simulink model "convertidor_pid_electrolizador"  (R2021a)
settings: Solver=VariableStepAuto  StartTime=0.0  StopTime=10  RelTol=1e-1
undefined symbols (not defined in the file): magnitude
libraries: spsSeriesRLCBranchLib x9, spsCurrentMeasurementLib x3, spsDiodeLib x3, simulink x3, spsGroundLib x2, spsMosfetLib x2, spsControlledVoltageSourceLib x1, pid_lib x1, spsDCVoltageSourceLib x1, spsVoltageMeasurementLib x1, spspowerguiLib x1
settings Model: Creator=Usuario  LastModifiedBy=Usuario

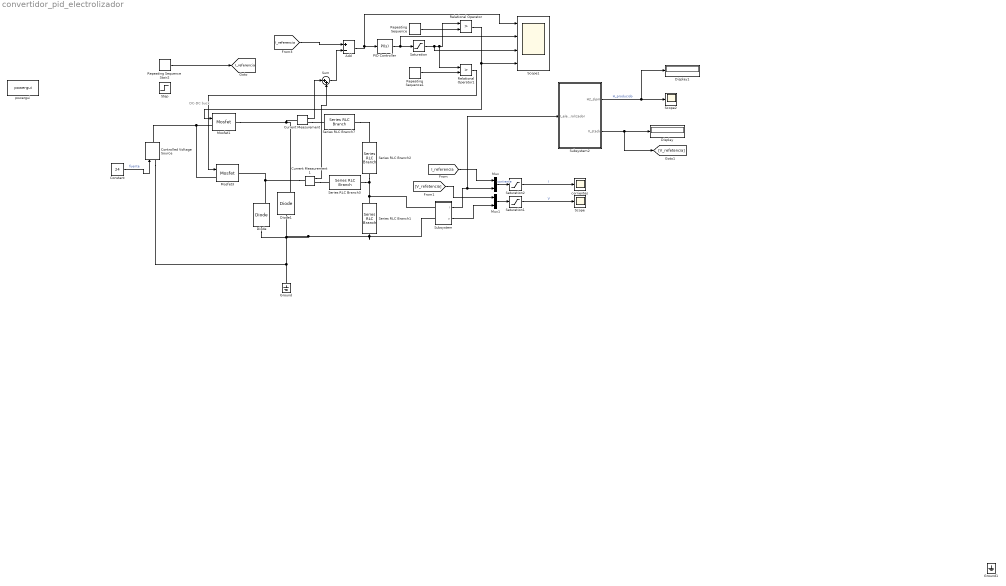
== system convertidor_pid_electrolizador ==
  note: DC-DC buck
  Add : Sum  Inputs=+-
  Constant : Constant  Value=24
  Controlled Voltage Source : spsControlledVoltageSourceLib/Controlled Voltage Source  Initialize=on  Source_Type=DC  Amplitude=10  Phase=0  Frequency=0  Measurements=None
  Current Measurement : spsCurrentMeasurementLib/Current Measurement  PhasorSimulation=off  OutputType=Complex  PSBequivalent=0
  Current Measurement1 : spsCurrentMeasurementLib/Current Measurement  PhasorSimulation=off  OutputType=Complex  PSBequivalent=0
  Diode : spsDiodeLib/Diode  Ron=0.001  Lon=0  Vf=0.8  IC=0  UseSnubber=0  Rs=500  Cs=250e-9  Measurements=on
  Diode1 : spsDiodeLib/Diode  Ron=0.001  Lon=0  Vf=0.8  IC=0  UseSnubber=0  Rs=500  Cs=250e-9  Measurements=on
  Display : Display
  Display1 : Display
  Ground : spsGroundLib/Ground  LConnTagsString=a
  Ground1 : spsGroundLib/Ground  LConnTagsString=a
  Mosfet1 : spsMosfetLib/Mosfet  Ron=0.001  Lon=0  Rd=0.01  Vfd=0  IC=0  Rs=1e5  Cs=inf  Measurements=off
  Mosfet3 : spsMosfetLib/Mosfet  Ron=0.001  Lon=0  Rd=0.01  Vfd=0  IC=0  Rs=1e5  Cs=inf  Measurements=off
  Mux : Mux  Inputs=2
  Mux1 : Mux  Inputs=2
  PID Controller : pid_lib/PID Controller  Controller=PI  Form=Parallel  TimeDomain=Continuous-time  UseExternalTs=off  SampleTime=-1  IntegratorMethod=Forward Euler  FilterMethod=Forward Euler  ControllerParametersSource=internal  P=7.85  I=261.799  D=1  UseFilter=on  N=1436119.989540  TunerSelectOption=Transfer Function Based (PID Tuner App)  InitialConditionSource=internal  InitialConditionForIntegrator=0  InitialConditionForFilter=0  DifferentiatorICPrevScaledInput=0  ExternalReset=none  TrackingMode=off  Kt=1  LimitOutput=off  SatLimitsSource=internal  UpperSaturationLimit=inf  LowerSaturationLimit=-inf  LinearizeAsGain=on  AntiWindupMode=none  Kb=1  POutMin=[]  POutMax=[]  IOutMin=[]  IOutMax=[]  DOutMin=[]  DOutMax=[]  NOutMin=[]  NOutMax=[]  SumOutMin=[]  SumOutMax=[]  SaturationOutMin=[]  SaturationOutMax=[]  PParamMin=[]  PParamMax=[]  IParamMin=[]  IParamMax=[]  DParamMin=[]  DParamMax=[]  NParamMin=[]  NParamMax=[]  KbParamMin=[]  KbParamMax=[]  KtParamMin=[]  KtParamMax=[]  KbOutMin=[]  KbOutMax=[]  KtOutMin=[]  KtOutMax=[]  IntegratorOutMin=[]  IntegratorOutMax=[]  FilterOutMin=[]  FilterOutMax=[]  SumI1OutMin=[]  SumI1OutMax=[]  SumI2OutMin=[]  SumI2OutMax=[]  SumI3OutMin=[]  SumI3OutMax=[]  SumI4OutMin=[]  SumI4OutMax=[]  SumDOutMin=[]  SumDOutMax=[]  DifferentiatorOutMin=[]  DifferentiatorOutMax=[]  FilterDiffOutCoefMin=[]  FilterDiffOutCoefMax=[]  ReciprocalOutMin=[]  ReciprocalOutMax=[]  SumDenOutMin=[]  SumDenOutMax=[]  SumNumOutMin=[]  SumNumOutMax=[]  DivideOutMin=[]  DivideOutMax=[]  UdiffTsProdOutMin=[]  UdiffTsProdOutMax=[]  NTsProdOutMin=[]  NTsProdOutMax=[]  UintegralTsProdOutMin=[]  UintegralTsProdOutMax=[]  UngainTsProdOutMin=[]  UngainTsProdOutMax=[]  IntegratorContinuousStateAttributes=''  IntegratorStateMustResolveToSignalObject=off  IntegratorRTWStateStorageClass=Auto  FilterContinuousStateAttributes=''  FilterStateMustResolveToSignalObject=off  FilterRTWStateStorageClass=Auto  ParallelPVariant=InternalParameters  IdealPVariant=Disabled  IVariant=InternalParameters  DVariant=Disabled  IntegratorVariant=Continuous  SatVariant=Disabled  AWVariant=Passthrough  PCopyVariant=Disabled  TRVariant=Disabled  FdbkBlocksVariant=Forward  IdealPFdbkVariant=Disabled  SatFdbkVariant=Disabled  DerivativeFilterVariant=Disabled  NVariant=Disabled  NCopyVariant=Disabled_SignalSpec  FilterICVariant=Disabled  IntegratorICVariant=InternalICs  ExternalResetVariant=Disabled  TRSumVariant=Passthrough  SumFdbkVariant=Disabled  SumVariant=Sum_PI  TsampFilterVariant=InternalTs  TsampNgainVariant=Passthrough  TsampIntegralVariant=Passthrough  ExternalSaturationOutDataTypeStr=Inherit: Same as second input
  Relational Operator : RelationalOperator  Operator=>  OutDataTypeStr=boolean  RndMeth=Simplest
  Relational Operator1 : RelationalOperator  Operator=>  OutDataTypeStr=boolean  RndMeth=Simplest
  Repeating Sequence : simulink/Sources/Repeating Sequence  rep_seq_t=[0 0.0001]  rep_seq_y=[0 1]
  Repeating Sequence Stair2 : simulink/Sources/Repeating Sequence Stair  OutValues=[0.1 10 40 19 20.8]  tsamp=2  OutMin=[]  OutMax=[]  OutDataTypeStr=double  OutputDataTypeScalingMode=double  OutDataType=fixdt(0,8)  ConRadixGroup=Best Precision: Vector-wise  OutScaling=2^-12
  Repeating Sequence1 : simulink/Sources/Repeating Sequence  rep_seq_t=[0 0.0001]  rep_seq_y=[1 0]
  Saturation : Saturate  UpperLimit=0.95  LowerLimit=0.01
  Saturation1 : Saturate  UpperLimit=19  LowerLimit=0
  Saturation2 : Saturate  UpperLimit=100  LowerLimit=0
  Scope : Scope
  Scope1 : Scope  NumInputPorts=4
  Scope2 : Scope
  Series RLC Branch1 : spsSeriesRLCBranchLib/Series RLC Branch  LConnTagsString=__new0  RConnTagsString=__new0  BranchType=C  Resistance=0.01  Inductance=1e-3  SetiL0=off  InitialCurrent=0  Capacitance=21.55e-6  Setx0=off  InitialVoltage=0  Measurements=None
  Series RLC Branch2 : spsSeriesRLCBranchLib/Series RLC Branch  LConnTagsString=__new0  RConnTagsString=__new0  BranchType=C  Resistance=0.01  Inductance=1e-3  SetiL0=off  InitialCurrent=0  Capacitance=21.55e-6  Setx0=off  InitialVoltage=0  Measurements=None
  Series RLC Branch3 : spsSeriesRLCBranchLib/Series RLC Branch  LConnTagsString=__new0  RConnTagsString=__new0  BranchType=L  Resistance=0.001  Inductance=299.6e-6  SetiL0=off  InitialCurrent=0  Capacitance=1e-6  Setx0=off  InitialVoltage=0  Measurements=None
  Series RLC Branch7 : spsSeriesRLCBranchLib/Series RLC Branch  LConnTagsString=__new0  RConnTagsString=__new0  BranchType=L  Resistance=0.001  Inductance=299.6e-6  SetiL0=off  InitialCurrent=0  Capacitance=1e-6  Setx0=off  InitialVoltage=0  Measurements=None
  Step : Step  Time=0.5  After=40  SampleTime=0
  Subsystem : Subsystem
  Subsystem2 : Subsystem
  Sum : Sum  Inputs=|++
  corrientes : Scope
  powergui : spspowerguiLib/powergui  Priority=1  SimulationMode=Discrete  SampleTime=1e-5  frequency=60  Iterations=50  frequencyindice=0  Pbase=100e6  ErrMax=1e-4  UnitsV=kV  UnitsW=MW  buscounter=0  FunctionMessages=off  echomessages=off  EnableUseOfTLC=off  CurrentSourceSwitches=off  DisableSnubberDevices=off  DisableRonSwitches=off  DisableVfSwitches=off  DisplayEquations=off  AutomaticDiscreteSolvers=off  SolverType=Tustin/Backward Euler (TBE)  Interpol=off  ExternalGateDelay=off  methode=off  Ts=100  x0status=blocks  SPID=on  SwTol=0  HookPort=off  NonlinearTolerance=1e-4  nMaxIteration=100  ContinueOnMaxIteration=off  RestoreLinks=warning  ResistiveCurrentMeasurement=off  Frange=[0:2:500]  Ylog=off  Xlog=on  ShowGrid=off  save=off  variable=ZData  structure=0  ZoomFFT=off  StartTime=0.0  cycles=1  DisplayStyle=1  fundamental=60  FreqAxis=off  MaxFrequency=1000  frequencyindicesteady=1  RmsSteady=1  display=off
  tag scope: I_referencia=global
  wires:
  Constant/1 -> Controlled Voltage Source/1  "fuente"
  Mux/1 -> Saturation2/1  "coriiente"
  Mux1/1 -> Saturation1/1
  Saturation1/1 -> Scope/1  "V"
  Saturation2/1 -> corrientes/1  "I"
  Subsystem2/2(V_stack) -> [V_refetencia], Display/1
  Subsystem/2(v) -> Mux1/2
  [I_referencia] -> Mux/1
  [V_refetencia] -> Mux1/1
  Current Measurement/1 -> Sum/1
  Current Measurement1/1 -> Sum/2
  [I_referencia] -> Add/1
  Add/1 -> Scope1/1, PID Controller/1
  PID Controller/1 -> Scope1/2, Saturation/1
  Saturation/1 -> Scope1/3, Relational Operator1/1, Relational Operator/1
  Repeating Sequence/1 -> Relational Operator/2
  Repeating Sequence1/1 -> Relational Operator1/2
  Relational Operator1/1 -> Mosfet3/1
  Relational Operator/1 -> Scope1/4, Mosfet1/1
  Subsystem/1(i) -> Subsystem2/1(I_electrolizador), Mux/2
  Subsystem2/1(H2_slpm) -> Display1/1, Scope2/1  "H_producido"
  Repeating Sequence Stair2/1 -> [I_referencia]
  Sum/1 -> Add/2
  connections:
  Series RLC Branch7/RConn1 -- Series RLC Branch2/LConn1
  Controlled Voltage Source/RConn1 -- Mosfet3/LConn1 -- Mosfet1/LConn1
  Current Measurement1/LConn1 -- Mosfet3/RConn1 -- Diode/RConn1
  Diode1/LConn1 -- Subsystem/LConn2 -- Series RLC Branch1/RConn1 -- Diode/LConn1 -- Controlled Voltage Source/LConn1 -- Ground/LConn1
  Mosfet1/RConn1 -- Diode1/RConn1 -- Current Measurement/LConn1
  Series RLC Branch3/RConn1 -- Subsystem/LConn1 -- Series RLC Branch1/LConn1 -- Series RLC Branch2/RConn1
  Current Measurement/RConn1 -- Series RLC Branch7/LConn1
  Current Measurement1/RConn1 -- Series RLC Branch3/LConn1

== system convertidor_pid_electrolizador/Subsystem ==
  Current Measurement : spsCurrentMeasurementLib/Current Measurement  PhasorSimulation=off  OutputType=Complex  PSBequivalent=0
  DC Voltage Source : spsDCVoltageSourceLib/DC Voltage Source  Amplitude=1.45*5  Measurements=None
  Diode : spsDiodeLib/Diode  Ron=0.001  Lon=0  Vf=0.8  IC=0  UseSnubber=0  Rs=500  Cs=250e-9  Measurements=off
  R.act : spsSeriesRLCBranchLib/Series RLC Branch  LConnTagsString=__new0  RConnTagsString=__new0  BranchType=R  Resistance=0.04  Inductance=1e-3  SetiL0=off  InitialCurrent=0  Capacitance=1e-6  Setx0=off  InitialVoltage=0  Measurements=None
  R.con : spsSeriesRLCBranchLib/Series RLC Branch  LConnTagsString=__new0  RConnTagsString=__new0  BranchType=R  Resistance=0.009  Inductance=1e-3  SetiL0=off  InitialCurrent=0  Capacitance=1e-6  Setx0=off  InitialVoltage=0  Measurements=None
  R.ohm : spsSeriesRLCBranchLib/Series RLC Branch  LConnTagsString=__new0  RConnTagsString=__new0  BranchType=R  Resistance=0.06  Inductance=1e-3  SetiL0=off  InitialCurrent=0  Capacitance=1e-6  Setx0=off  InitialVoltage=0  Measurements=None
  Series RLC Branch1 : spsSeriesRLCBranchLib/Series RLC Branch  LConnTagsString=__new0  RConnTagsString=__new0  BranchType=C  Resistance=1  Inductance=1e-3  SetiL0=off  InitialCurrent=0  Capacitance=0.02  Setx0=off  InitialVoltage=0  Measurements=None
  Series RLC Branch3 : spsSeriesRLCBranchLib/Series RLC Branch  LConnTagsString=__new0  RConnTagsString=__new0  BranchType=C  Resistance=1  Inductance=1e-3  SetiL0=off  InitialCurrent=0  Capacitance=437  Setx0=off  InitialVoltage=0  Measurements=None
  Voltage Measurement : spsVoltageMeasurementLib/Voltage Measurement  PhasorSimulation=off  OutputType=Complex  PSBequivalent=0
  + : PMIOPort  Side=Left
  - : PMIOPort  Port=2  Side=Left
  i : Outport
  v : Outport  Port=2
  wires:
  Current Measurement/1 -> i/1
  Voltage Measurement/1 -> v/1
  connections:
  R.ohm/RConn1 -- R.act/LConn1 -- Series RLC Branch1/LConn1
  Voltage Measurement/LConn1 -- Current Measurement/RConn1 -- DC Voltage Source/RConn1
  Series RLC Branch3/LConn1 -- Series RLC Branch1/RConn1
  R.ohm/LConn1 -- DC Voltage Source/LConn1
  Diode/RConn1 -- Current Measurement/LConn1
  Diode/LConn1 -- +/RConn1
  R.act/RConn1 -- R.con/LConn1
  R.con/RConn1 -- Voltage Measurement/LConn2 -- Series RLC Branch3/RConn1 -- -/RConn1

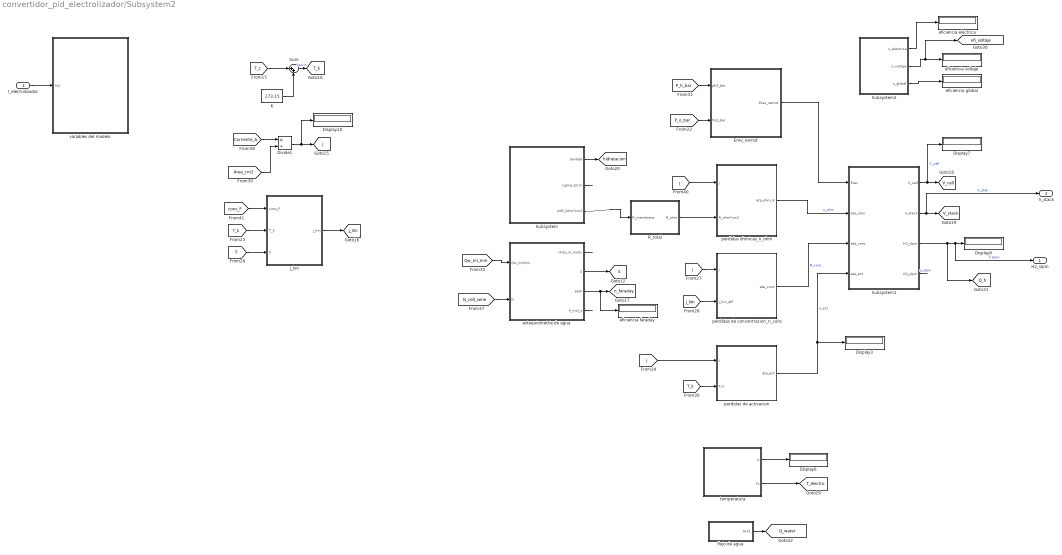
== system convertidor_pid_electrolizador/Subsystem2 ==
  I_electrolizador : Inport
  Display{3,6..8,10} (5 alike) : Display
  Divide1 : Product  Inputs=*/
  Erev_nernst : Subsystem
  K : Constant  Value=273.15
  R_total : Subsystem
  Subsystem : Subsystem
  Subsystem1 : Subsystem
  Subsystem2 : Subsystem
  Sum : Sum  Inputs=|++
  eficiencia electrica : Display
  eficiencia faraday : Display
  eficiencia global : Display
  eficiencia voltaje : Display
  estequiometria de agua : Subsystem
  flujo de agua : Subsystem
  j_lim : Subsystem
  perdidas de activacion : Subsystem
  perdidas de concentracion_n_conc : Subsystem
  perdidas ohmicas_n_ohm : Subsystem
  temperatura : Subsystem
  variables del modelo : Subsystem
  H2_slpm : Outport
  V_stack : Outport  Port=2
  tag scope: Q_h=global, Q_water=global, S=global, T_electro=global, T_k=global, V_cell=global, V_stack=global, efi_voltaje=global, hidratacion=global, j=global, j_lim=global, n_faraday=global
  wires:
  [T_k] -> j_lim/2(T_k)
  R_total/1(R_ohm) -> perdidas ohmicas_n_ohm/2(R_ohm*cm2)
  Subsystem2/2(n_voltaje) -> [efi_voltaje], eficiencia voltaje/1
  Subsystem1/3(H2_slpm) -> [Q_h], H2_slpm/1, Display8/1  "h slpm"
  Subsystem1/1(V_cell) -> Display7/1, [V_cell]  "V_cell"
  [j_lim] -> perdidas de concentracion_n_conc/2(j_lim_eff)
  [Qw_ml_min] -> estequiometria de agua/1(Qw_ml/min)
  [N_cell_serie] -> estequiometria de agua/2(N)
  Subsystem2/1(n_electrica) -> eficiencia electrica/1
  Erev_nernst/1(Erev_nernst) -> Subsystem1/1(Erev)
  temperatura/2(ºc) -> [T_electro]
  perdidas ohmicas_n_ohm/1(eta_ohm_V) -> Subsystem1/2(eta_ohm)  "n_ohm"
  Subsystem2/3(n_global) -> eficiencia global/1
  perdidas de activacion/1(eta_act) -> Subsystem1/4(eta_act), Display3/1  "n_act"
  [j] -> perdidas ohmicas_n_ohm/1(j)
  estequiometria de agua/3(etaF) -> eficiencia faraday/1, [n_faraday]
  j_lim/1(j_lim) -> [j_lim]
  flujo de agua/1(Out1) -> [Q_water]
  Subsystem/1(lambda) -> [hidratacion]
  [S] -> j_lim/3(S)
  K/1 -> Sum/2
  Sum/1 -> [T_k]  "kelvin"
  estequiometria de agua/1(nh2o_in_mol/s) -> ?
  [cons_F] -> j_lim/1(cons_F)
  [Area_cm2] -> Divide1/2
  temperatura/1(K) -> Display6/1
  estequiometria de agua/4(h_mol_s) -> ?
  Subsystem1/2(V_stack) -> V_stack/1, [V_stack]  "V_stak"
  [P_o_bar] -> Erev_nernst/2(Po2_bar)
  perdidas de concentracion_n_conc/1(eta_conc) -> Subsystem1/3(eta_conc)  "N_conc"
  [P_h_bar] -> Erev_nernst/1(ph2_bar)
  [j] -> perdidas de activacion/1(j)
  Divide1/1 -> Display10/1, [j]
  [j] -> perdidas de concentracion_n_conc/1(j)
  estequiometria de agua/2(S) -> [S]
  [T_k] -> perdidas de activacion/2(T_k)
  [T_c] -> Sum/1
  [Corriente_A] -> Divide1/1
  Subsystem/3(ASR_Ohm*cm2) -> R_total/1(R_membrana)
  Subsystem/2(sigma_S/cm) -> ?
  Subsystem1/4(O2_slpm) -> ?  "o_slpm"
  I_electrolizador/1 -> variables del modelo/1(In1)

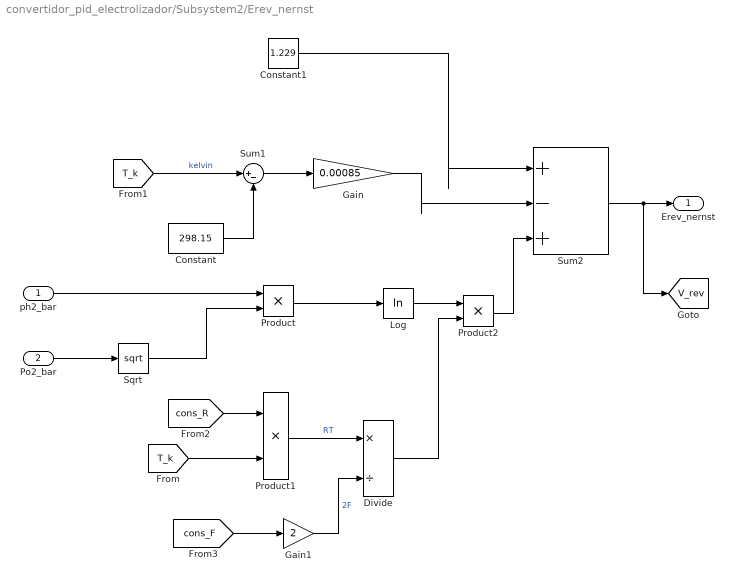
== system convertidor_pid_electrolizador/Subsystem2/Erev_nernst ==
  ph2_bar : Inport
  Po2_bar : Inport  Port=2
  Constant : Constant  Value=298.15
  Constant1 : Constant  Value=1.229
  Divide : Product  Inputs=*/
  Gain : Gain  Gain=0.00085
  Gain1 : Gain  Gain=2
  Log : Math  Operator=log  SaturateOnIntegerOverflow=on
  Product : Product
  Product1 : Product
  Product2 : Product
  Sqrt : Sqrt  SaturateOnIntegerOverflow=on
  Sum1 : Sum  Inputs=|+-
  Sum2 : Sum  Inputs=|+-+
  Erev_nernst : Outport
  tag scope: V_rev=global
  wires:
  [T_k] -> Sum1/1  "kelvin"
  Constant/1 -> Sum1/2
  Sum1/1 -> Gain/1
  Po2_bar/1 -> Sqrt/1
  ph2_bar/1 -> Product/1
  Sqrt/1 -> Product/2
  Constant1/1 -> Sum2/1
  Gain/1 -> Sum2/2
  Product/1 -> Log/1
  [T_k] -> Product1/2
  [cons_R] -> Product1/1
  Product1/1 -> Divide/1  "RT"
  [cons_F] -> Gain1/1
  Gain1/1 -> Divide/2  "2F"
  Log/1 -> Product2/1
  Divide/1 -> Product2/2
  Product2/1 -> Sum2/3
  Sum2/1 -> [V_rev], Erev_nernst/1

== system convertidor_pid_electrolizador/Subsystem2/R_total ==
  R_membrana : Inport
  Sum : Sum  Inputs=|++
  R_ohm : Outport
  wires:
  Sum/1 -> R_ohm/1
  R_membrana/1 -> Sum/1
  [R_contacto] -> Sum/2

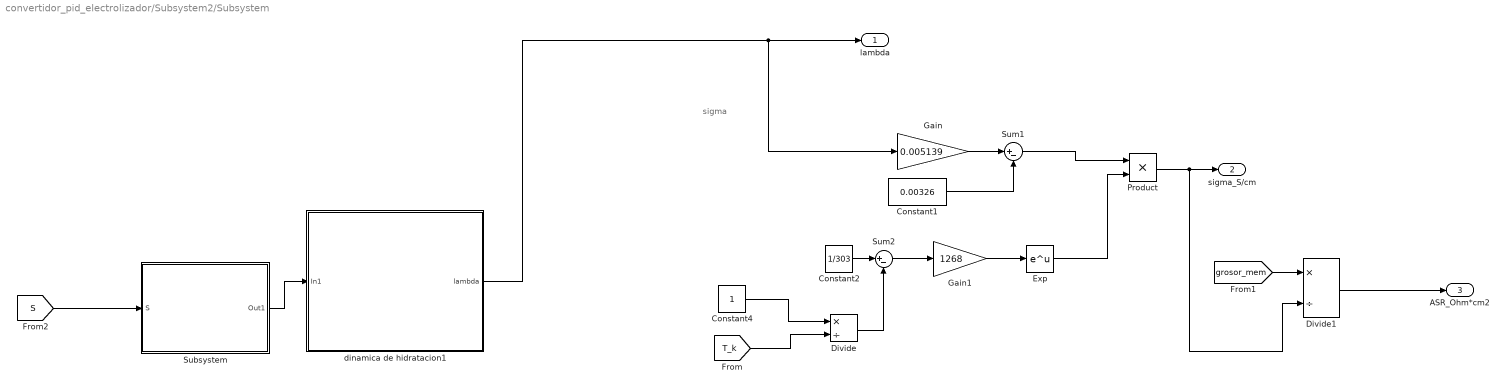
== system convertidor_pid_electrolizador/Subsystem2/Subsystem ==
  note: sigma
  Constant1 : Constant  Value=0.00326
  Constant2 : Constant  Value=1/303
  Constant4 : Constant
  Divide : Product  Inputs=*/
  Divide1 : Product  Inputs=*/
  Exp : Math  SaturateOnIntegerOverflow=on
  Gain : Gain  Gain=0.005139
  Gain1 : Gain  Gain=1268
  Product : Product
  Subsystem : Subsystem
  Sum1 : Sum  Inputs=|+-
  Sum2 : Sum  Inputs=|+-
  dinamica de hidratacion1 : Subsystem
  lambda : Outport
  sigma_S/cm : Outport  Port=2
  ASR_Ohm*cm2 : Outport  Port=3
  wires:
  [grosor_mem] -> Divide1/1
  [T_k] -> Divide/2
  Sum2/1 -> Gain1/1
  Exp/1 -> Product/2
  Divide/1 -> Sum2/2
  Constant1/1 -> Sum1/2
  Gain/1 -> Sum1/1
  Gain1/1 -> Exp/1
  Constant4/1 -> Divide/1
  Constant2/1 -> Sum2/1
  Sum1/1 -> Product/1
  dinamica de hidratacion1/1(lambda) -> Gain/1, lambda/1
  Subsystem/1(Out1) -> dinamica de hidratacion1/1(In1)
  [S] -> Subsystem/1(S)
  Divide1/1 -> ASR_Ohm*cm2/1
  Product/1 -> Divide1/2, sigma_S/cm/1

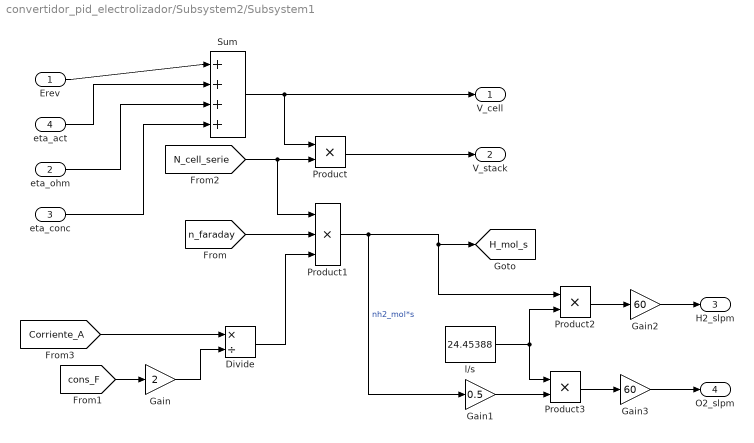
== system convertidor_pid_electrolizador/Subsystem2/Subsystem1 ==
  Erev : Inport
  eta_ohm : Inport  Port=2
  eta_conc : Inport  Port=3
  eta_act : Inport  Port=4
  Divide : Product  Inputs=*/
  Gain : Gain  Gain=2
  Gain1 : Gain  Gain=0.5
  Gain2 : Gain  Gain=60
  Gain3 : Gain  Gain=60
  Product : Product
  Product1 : Product  Inputs=3
  Product2 : Product
  Product3 : Product
  Sum : Sum  Inputs=|++++
  l/s : Constant  Value=24.45388
  V_cell : Outport
  V_stack : Outport  Port=2
  H2_slpm : Outport  Port=3
  O2_slpm : Outport  Port=4
  tag scope: H_mol_s=global
  wires:
  Erev/1 -> Sum/1
  eta_act/1 -> Sum/2
  eta_ohm/1 -> Sum/3
  eta_conc/1 -> Sum/4
  Sum/1 -> Product/1, V_cell/1
  [N_cell_serie] -> Product1/1, Product/2
  Product/1 -> V_stack/1
  Product1/1 -> Gain1/1, [H_mol_s], Product2/1  "nh2_mol*s"
  [n_faraday] -> Product1/2
  [cons_F] -> Gain/1
  [Corriente_A] -> Divide/1
  Gain/1 -> Divide/2
  Divide/1 -> Product1/3
  Gain1/1 -> Product3/2
  l/s/1 -> Product2/2, Product3/1
  Product2/1 -> Gain2/1
  Product3/1 -> Gain3/1
  Gain2/1 -> H2_slpm/1
  Gain3/1 -> O2_slpm/1

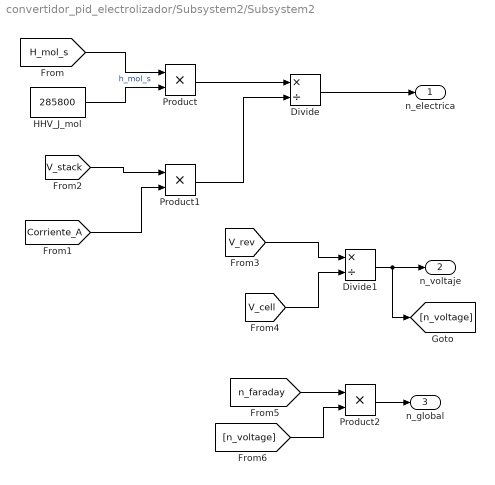
== system convertidor_pid_electrolizador/Subsystem2/Subsystem2 ==
  Divide : Product  Inputs=*/
  Divide1 : Product  Inputs=*/
  HHV_J_mol : Constant  Value=285800
  Product : Product
  Product1 : Product
  Product2 : Product
  n_electrica : Outport
  n_voltaje : Outport  Port=2
  n_global : Outport  Port=3
  wires:
  Divide/1 -> n_electrica/1
  Product/1 -> Divide/1
  Product1/1 -> Divide/2
  [H_mol_s] -> Product/1  "h_mol_s"
  HHV_J_mol/1 -> Product/2
  [V_stack] -> Product1/1
  [Corriente_A] -> Product1/2
  Divide1/1 -> [n_voltage], n_voltaje/1
  [V_cell] -> Divide1/2
  [V_rev] -> Divide1/1
  Product2/1 -> n_global/1
  [n_faraday] -> Product2/1
  [n_voltage] -> Product2/2

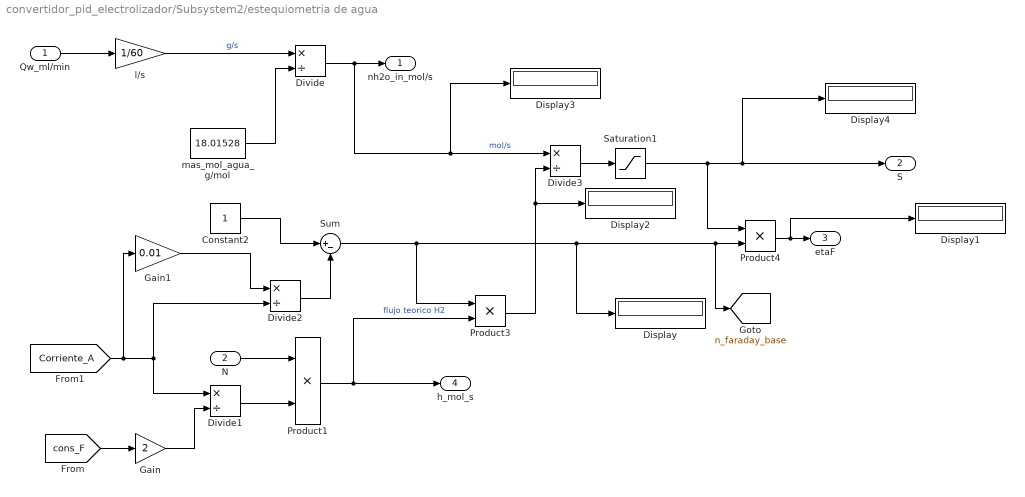
== system convertidor_pid_electrolizador/Subsystem2/estequiometria de agua ==
  Qw_ml/min : Inport
  N : Inport  Port=2
  Constant2 : Constant
  Display{,1..4} (5 alike) : Display
  Divide{,1..3} (4 alike) : Product  Inputs=*/
  Gain : Gain  Gain=2
  Gain1 : Gain  Gain=0.01
  Product1 : Product
  Product3 : Product
  Product4 : Product
  Saturation1 : Saturate  UpperLimit=1  LowerLimit=0
  Sum : Sum  Inputs=|+-
  l/s : Gain  Gain=1/60
  mas_mol_agua_g/mol : Constant  Value=18.01528
  nh2o_in_mol/s : Outport
  S : Outport  Port=2
  etaF : Outport  Port=3
  h_mol_s : Outport  Port=4
  tag scope: n_faraday_base=global
  wires:
  l/s/1 -> Divide/1  "g/s"
  mas_mol_agua_g/mol/1 -> Divide/2
  Divide/1 -> Display3/1, Divide3/1, nh2o_in_mol/s/1  "mol/s"
  [cons_F] -> Gain/1
  Gain/1 -> Divide1/2
  Divide1/1 -> Product1/2
  [Corriente_A] -> Gain1/1, Divide2/2, Divide1/1
  Constant2/1 -> Sum/1
  Divide2/1 -> Sum/2
  Sum/1 -> Product3/1, Display/1, [n_faraday_base], Product4/2
  Product1/1 -> h_mol_s/1, Product3/2  "flujo teorico H2"
  Divide3/1 -> Saturation1/1
  Product3/1 -> Display2/1, Divide3/2
  Product4/1 -> Display1/1, etaF/1
  Saturation1/1 -> Product4/1, Display4/1, S/1
  Qw_ml/min/1 -> l/s/1
  Gain1/1 -> Divide2/1
  N/1 -> Product1/1

== system convertidor_pid_electrolizador/Subsystem2/flujo de agua ==
  Display : Display
  Divide : Product  Inputs=*/
  Gain : Gain  Gain=18.015
  Gain1 : Gain  Gain=60
  Gain2 : Gain  Gain=2
  Product : Product
  Product1 : Product
  Out1 : Outport
  wires:
  Gain/1 -> Gain1/1
  Gain1/1 -> Display/1, Out1/1
  [cons_F] -> Gain2/1
  [n_faraday_base] -> Product/1
  [Corriente_A] -> Product/2
  Product/1 -> Divide/1
  Gain2/1 -> Divide/2
  Divide/1 -> Product1/2  "mol/s"
  Product1/1 -> Gain/1
  [N_cell_serie] -> Product1/1

== system convertidor_pid_electrolizador/Subsystem2/j_lim ==
  cons_F : Inport
  T_k : Inport  Port=2
  S : Inport  Port=3
  Constant : Constant  Value=2
  Constant5 : Constant  Value=298
  Divide : Product  Inputs=*/
  Divide1 : Product  Inputs=*/
  Dref : Constant  Value=2e-6
  Power : Math  Operator=pow  SaturateOnIntegerOverflow=on
  Product : Product  Inputs=5
  Product1 : Product
  concentracion de agua _mol_cm3 : Constant  Value=0.0555
  espesor difucion : Constant  Value=0.01
  m : Constant  Value=1.5
  j_lim : Outport
  wires:
  Constant/1 -> Product/1
  espesor difucion/1 -> Divide/2
  cons_F/1 -> Product/2
  Product/1 -> Divide/1
  Divide/1 -> j_lim/1
  Product1/1 -> Product/3  "difucion del agua"
  Dref/1 -> Product1/1
  Power/1 -> Product1/2
  Divide1/1 -> Power/1
  m/1 -> Power/2
  T_k/1 -> Divide1/1
  Constant5/1 -> Divide1/2
  concentracion de agua _mol_cm3/1 -> Product/4
  S/1 -> Product/5

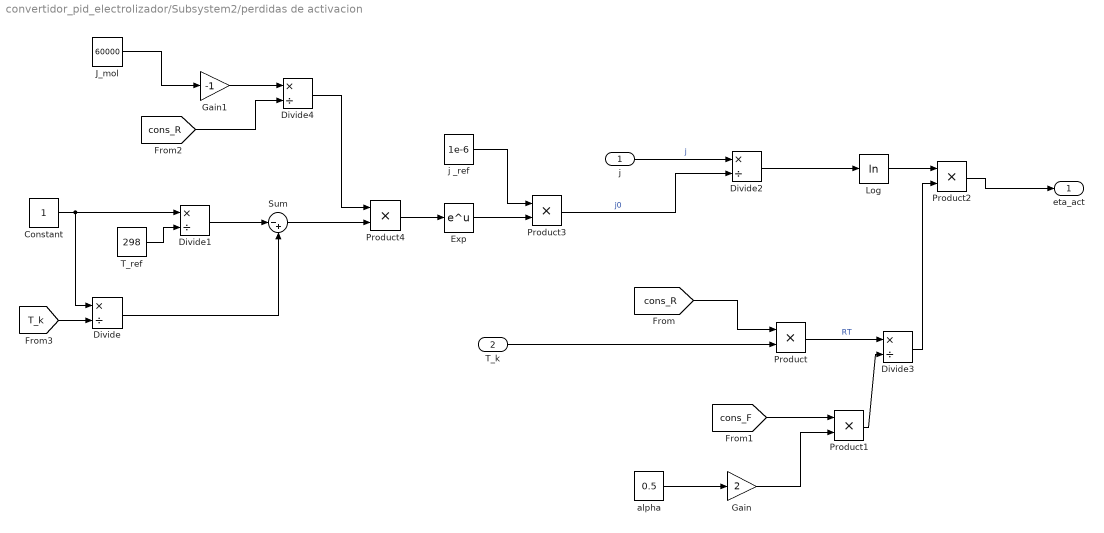
== system convertidor_pid_electrolizador/Subsystem2/perdidas de activacion ==
  j : Inport
  T_k : Inport  Port=2
  Constant : Constant
  Divide{,1..4} (5 alike) : Product  Inputs=*/
  Exp : Math  SaturateOnIntegerOverflow=on
  Gain : Gain  Gain=2
  Gain1 : Gain  Gain=-1
  J_mol : Constant  Value=60000
  Log : Math  Operator=log  SaturateOnIntegerOverflow=on
  Product{,1..4} (5 alike) : Product
  Sum : Sum  Inputs=|-+
  T_ref : Constant  Value=298
  alpha : Constant  Value=0.5
  j _ref : Constant  Value=1e-6
  eta_act : Outport
  wires:
  j/1 -> Divide2/1  "j"
  Product3/1 -> Divide2/2  "j0"
  Divide2/1 -> Log/1
  Log/1 -> Product2/1
  [cons_R] -> Product/1
  T_k/1 -> Product/2
  [cons_F] -> Product1/1
  Product1/1 -> Divide3/2
  Product/1 -> Divide3/1  "RT"
  Divide3/1 -> Product2/2
  Product2/1 -> eta_act/1
  Gain/1 -> Product1/2
  alpha/1 -> Gain/1
  j _ref/1 -> Product3/1
  Constant/1 -> Divide/1, Divide1/1
  T_ref/1 -> Divide1/2
  Divide1/1 -> Sum/1
  Divide/1 -> Sum/2
  Sum/1 -> Product4/2
  Divide4/1 -> Product4/1
  Gain1/1 -> Divide4/1
  [cons_R] -> Divide4/2
  Product4/1 -> Exp/1
  Exp/1 -> Product3/2
  J_mol/1 -> Gain1/1
  [T_k] -> Divide/2

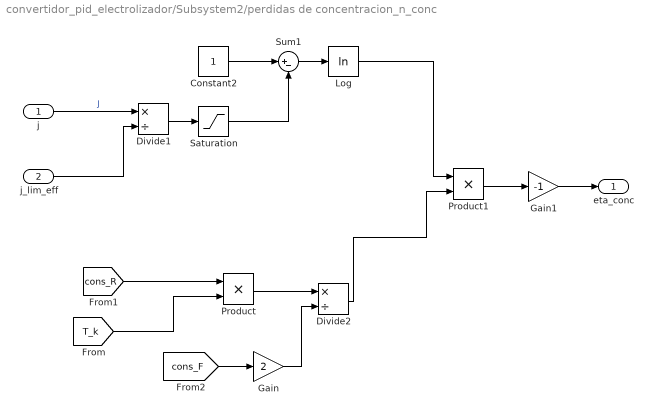
== system convertidor_pid_electrolizador/Subsystem2/perdidas de concentracion_n_conc ==
  j : Inport
  j_lim_eff : Inport  Port=2
  Constant2 : Constant
  Divide1 : Product  Inputs=*/
  Divide2 : Product  Inputs=*/
  Gain : Gain  Gain=2
  Gain1 : Gain  Gain=-1
  Log : Math  Operator=log  SaturateOnIntegerOverflow=on
  Product : Product
  Product1 : Product
  Saturation : Saturate  UpperLimit=0.999  LowerLimit=0
  Sum1 : Sum  Inputs=|+-
  eta_conc : Outport
  wires:
  j/1 -> Divide1/1  "J"
  j_lim_eff/1 -> Divide1/2
  Divide1/1 -> Saturation/1
  Constant2/1 -> Sum1/1
  Saturation/1 -> Sum1/2
  [cons_R] -> Product/1
  [cons_F] -> Gain/1
  Product/1 -> Divide2/1
  Gain/1 -> Divide2/2
  Sum1/1 -> Log/1
  Log/1 -> Product1/1
  Product1/1 -> Gain1/1
  [T_k] -> Product/2
  Divide2/1 -> Product1/2
  Gain1/1 -> eta_conc/1

== system convertidor_pid_electrolizador/Subsystem2/perdidas ohmicas_n_ohm ==
  j : Inport
  R_ohm*cm2 : Inport  Port=2
  Product : Product
  eta_ohm_V : Outport
  wires:
  j/1 -> Product/1  "J"
  Product/1 -> eta_ohm_V/1
  R_ohm*cm2/1 -> Product/2

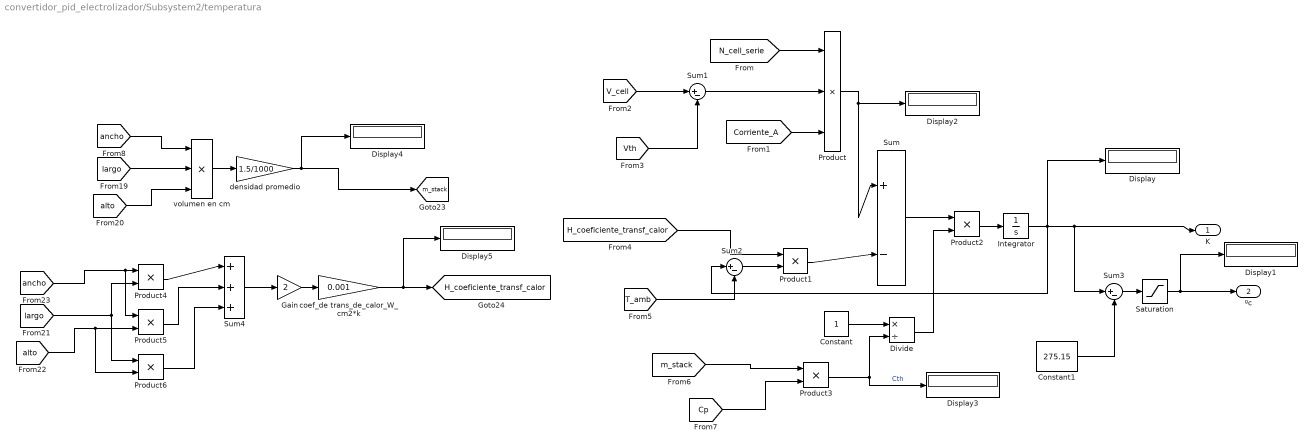
== system convertidor_pid_electrolizador/Subsystem2/temperatura ==
  Constant : Constant
  Constant1 : Constant  Value=275.15
  Display{,1..5} (6 alike) : Display
  Divide : Product  Inputs=*/
  Gain : Gain  Gain=2
  Integrator : Integrator
  Product : Product  Inputs=3
  Product{1..6} (6 alike) : Product
  Saturation : Saturate  UpperLimit=80  LowerLimit=10
  Sum{,1..3} (4 alike) : Sum  Inputs=|+-
  Sum4 : Sum  Inputs=|+++
  coef_de trans_de_calor_W_cm2*k : Gain  Gain=0.001
  densidad promedio : Gain  Gain=1.5/1000
  volumen en cm : Product  Inputs=3
  K : Outport
  ºc : Outport  Port=2
  tag scope: H_coeficiente_transf_calor=global, m_stack=global
  wires:
  Product/1 -> Display2/1, Sum/1
  [N_cell_serie] -> Product/1
  [Corriente_A] -> Product/3
  Sum1/1 -> Product/2
  [V_cell] -> Sum1/1
  [Vth] -> Sum1/2
  Product1/1 -> Sum/2
  Sum2/1 -> Product1/2
  [H_coeficiente_transf_calor] -> Product1/1
  [T_amb] -> Sum2/2
  Sum/1 -> Product2/1
  Divide/1 -> Product2/2
  Constant/1 -> Divide/1
  Product3/1 -> Display3/1, Divide/2  "Cth"
  [Cp] -> Product3/2
  [m_stack] -> Product3/1
  Constant1/1 -> Sum3/2
  Sum3/1 -> Saturation/1
  Product2/1 -> Integrator/1
  Integrator/1 -> Sum2/1, Sum3/1, K/1, Display/1
  Saturation/1 -> Display1/1, ºc/1
  Gain/1 -> coef_de trans_de_calor_W_cm2*k/1
  volumen en cm/1 -> densidad promedio/1
  Sum4/1 -> Gain/1
  Product5/1 -> Sum4/2
  [largo] -> volumen en cm/2
  [alto] -> volumen en cm/3
  [ancho] -> volumen en cm/1
  [alto] -> Product6/2, Product5/2
  [largo] -> Product6/1, Product4/2
  [ancho] -> Product5/1, Product4/1
  coef_de trans_de_calor_W_cm2*k/1 -> Display5/1, [H_coeficiente_transf_calor]
  Product4/1 -> Sum4/1
  densidad promedio/1 -> Display4/1, [m_stack]
  Product6/1 -> Sum4/3

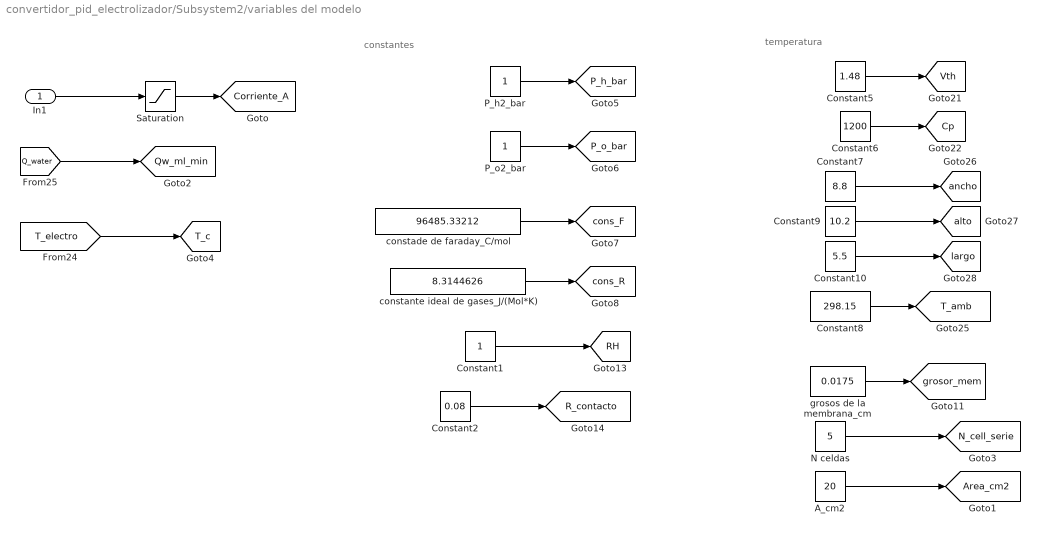
== system convertidor_pid_electrolizador/Subsystem2/variables del modelo ==
  note: constantes
  note: temperatura
  In1 : Inport
  A_cm2 : Constant  Value=20
  Constant1 : Constant
  Constant10 : Constant  Value=5.5
  Constant2 : Constant  Value=0.08
  Constant5 : Constant  Value=1.48
  Constant6 : Constant  Value=1200
  Constant7 : Constant  Value=8.8
  Constant8 : Constant  Value=298.15
  Constant9 : Constant  Value=10.2
  N celdas : Constant  Value=5
  P_h2_bar : Constant
  P_o2_bar : Constant
  Saturation : Saturate  UpperLimit=4000  LowerLimit=0.1
  constade de faraday_C/mol : Constant  Value=96485.33212
  constante ideal de gases_J/(Mol*K) : Constant  Value=8.3144626
  grosos de la membrana_cm : Constant  Value=0.0175
  tag scope: Area_cm2=global, Corriente_A=global, Cp=global, N_cell_serie=global, P_h_bar=global, P_o_bar=global, Qw_ml_min=global, RH=global, R_contacto=global, T_amb=global, T_c=global, Vth=global, alto=global, ancho=global, cons_F=global, cons_R=global, grosor_mem=global, largo=global
  wires:
  Constant6/1 -> [Cp]
  Constant7/1 -> [ancho]
  Constant5/1 -> [Vth]
  Constant9/1 -> [alto]
  Constant10/1 -> [largo]
  Constant8/1 -> [T_amb]
  [Q_water] -> [Qw_ml_min]
  In1/1 -> Saturation/1
  [T_electro] -> [T_c]
  Saturation/1 -> [Corriente_A]
  N celdas/1 -> [N_cell_serie]
  A_cm2/1 -> [Area_cm2]
  grosos de la membrana_cm/1 -> [grosor_mem]
  Constant1/1 -> [RH]
  P_h2_bar/1 -> [P_h_bar]
  P_o2_bar/1 -> [P_o_bar]
  constade de faraday_C/mol/1 -> [cons_F]
  constante ideal de gases_J/(Mol*K)/1 -> [cons_R]
  Constant2/1 -> [R_contacto]

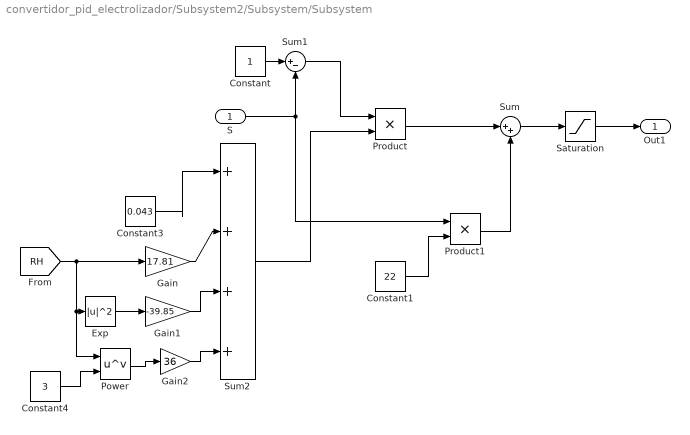
== system convertidor_pid_electrolizador/Subsystem2/Subsystem/Subsystem ==
  S : Inport
  Constant : Constant
  Constant1 : Constant  Value=22
  Constant3 : Constant  Value=0.043
  Constant4 : Constant  Value=3
  Exp : Math  Operator=magnitude^2  SaturateOnIntegerOverflow=on
  Gain : Gain  Gain=17.81
  Gain1 : Gain  Gain=-39.85
  Gain2 : Gain  Gain=36
  Power : Math  Operator=pow  SaturateOnIntegerOverflow=on
  Product : Product
  Product1 : Product
  Saturation : Saturate  UpperLimit=22  LowerLimit=0
  Sum : Sum  Inputs=|++
  Sum1 : Sum  Inputs=|+-
  Sum2 : Sum  Inputs=|++++
  Out1 : Outport
  wires:
  Product/1 -> Sum/1
  Product1/1 -> Sum/2
  Constant1/1 -> Product1/2
  Constant/1 -> Sum1/1
  Sum1/1 -> Product/1
  Sum2/1 -> Product/2
  S/1 -> Product1/1, Sum1/2
  Sum/1 -> Saturation/1
  Constant3/1 -> Sum2/1
  Gain1/1 -> Sum2/3
  Gain2/1 -> Sum2/4
  Gain/1 -> Sum2/2
  Exp/1 -> Gain1/1
  [RH] -> Power/1, Exp/1, Gain/1
  Power/1 -> Gain2/1
  Constant4/1 -> Power/2
  Saturation/1 -> Out1/1

== system convertidor_pid_electrolizador/Subsystem2/Subsystem/dinamica de hidratacion1 ==
  In1 : Inport
  Gain : Gain  Gain=1/0.5
  Integrator : Integrator
  Product1 : Product
  Product2 : Product
  Saturation : Saturate  UpperLimit=22  LowerLimit=0
  Sign : Signum
  Sum5 : Sum  Inputs=|+-
  Sum6 : Sum  Inputs=|++
  k_back : Constant
  k_drag : Constant  Value=0.2
  lambda : Outport
  wires:
  k_back/1 -> Product1/1
  Sign/1 -> Product2/1
  Product1/1 -> Gain/1
  k_drag/1 -> Product2/2
  Product2/1 -> Sum6/2
  Sum5/1 -> Product1/2
  Sum6/1 -> Integrator/1
  In1/1 -> Sum5/1
  Integrator/1 -> Sum5/2, Saturation/1
  Gain/1 -> Sum6/1
  [Corriente_A] -> Sign/1
  Saturation/1 -> lambda/1
